simulink model "pos_dvig"  (R2012b)
settings: Solver=ode23tb  StartTime=0.0  StopTime=10  RelTol=1e-3
values from neighbouring files (symbols this model uses):
  J = Jr + Jh    (= 0.0002754438)    [Parameters.m]
  k = 1/(3*R)    (= 0.537634408602)    [Parameters.m]
  ki = 25.5e-3*1/2    (= 0.01275)    [Parameters.m]
  KV = 374    [Parameters.m]
  kw = 30/(KV*pi)*1/2    (= 0.0127664392854)    [Parameters.m]
  P = 8    [Parameters.m]
  Te = L/R    (= 0.000451612903226)    [Parameters.m]
  U = 12    [Parameters.m]
undefined symbols (not defined in the file or in its folder): trapezoid
libraries: simulink x1
settings Model: Creator=botva  LastModifiedBy=botva

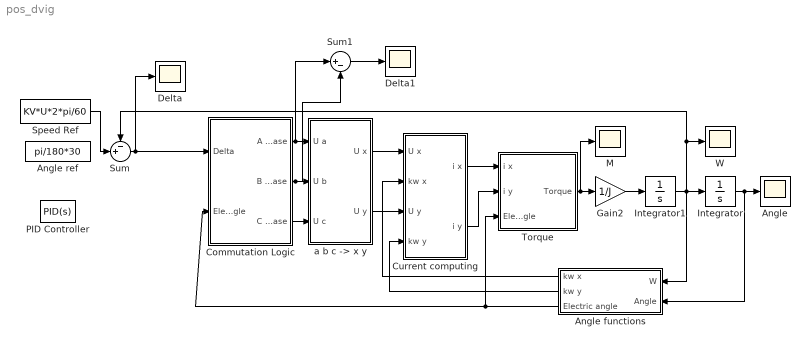
== system pos_dvig ==
  Angle : Scope
      settings: TimeRange=0.06  YMin=-500  YMax=500  DataFormat=Structure
  Angle functions : Subsystem
  Angle ref : Constant  Value=pi/180*30
  Commutation Logic : Subsystem
  Current computing : Subsystem
  Delta : Scope
      settings: TimeRange=0.06  YMin=-500  YMax=500  DataFormat=Structure
  Delta1 : Scope
      settings: TimeRange=0.06  YMin=-12.5  YMax=12.5  SaveName=ScopeData3  DataFormat=Structure
  Gain2 : Gain  Gain=1/J
  Integrator : Integrator
  Integrator1 : Integrator
  M : Scope
      settings: TimeRange=0.06  YMin=-0.025  YMax=0.25  SaveName=ScopeData2  DataFormat=Structure
  PID Controller : simulink/Continuous/PID Controller  Controller=PID  TimeDomain=Continuous-time  SampleTime=1  IntegratorMethod=Forward Euler  FilterMethod=Forward Euler  Form=Parallel  P=0.123357811480852  I=0.544614803683012  D=0.00224722047388112  N=3018.52790886393  InitialConditionSource=internal  InitialConditionForIntegrator=0  InitialConditionForFilter=0  ExternalReset=none  LimitOutput=off  UpperSaturationLimit=inf  LowerSaturationLimit=-inf  LinearizeAsGain=on  AntiWindupMode=none  Kb=1  TrackingMode=off  Kt=1  PParamMin=[]  PParamMax=[]  IParamMin=[]  IParamMax=[]  DParamMin=[]  DParamMax=[]  NParamMin=[]  NParamMax=[]  KbParamMin=[]  KbParamMax=[]  KtParamMin=[]  KtParamMax=[]  POutMin=[]  POutMax=[]  IOutMin=[]  IOutMax=[]  DOutMin=[]  DOutMax=[]  NOutMin=[]  NOutMax=[]  KbOutMin=[]  KbOutMax=[]  KtOutMin=[]  KtOutMax=[]  IntegratorOutMin=[]  IntegratorOutMax=[]  FilterOutMin=[]  FilterOutMax=[]  SumOutMin=[]  SumOutMax=[]  SumI1OutMin=[]  SumI1OutMax=[]  SumI2OutMin=[]  SumI2OutMax=[]  SumI3OutMin=[]  SumI3OutMax=[]  SumDOutMin=[]  SumDOutMax=[]  SaturationOutMin=[]  SaturationOutMax=[]  IntegratorContinuousStateAttributes=''  IntegratorStateMustResolveToSignalObject=off  IntegratorRTWStateStorageClass=Auto  FilterContinuousStateAttributes=''  FilterStateMustResolveToSignalObject=off  FilterRTWStateStorageClass=Auto
  Speed Ref : Constant  Value=KV*U*2*pi/60
  Sum : Sum  Inputs=-+|
  Sum1 : Sum  Inputs=|+-
  Torque : Subsystem
  W : Scope
      settings: TimeRange=0.06  YMin=469.973  YMax=470  SaveName=ScopeData6  DataFormat=Structure
  "a b c -> x y" : Subsystem
  wires:
  Integrator1/1 -> Angle functions/1(W), W/1, Sum/1, Integrator/1
  Integrator/1 -> Angle/1, Angle functions/2(Angle)
  "a b c -> x y"/1(U x) -> Current computing/1(U x)
  Gain2/1 -> Integrator1/1
  Angle functions/3(Electric angle) -> Torque/3(Electric angle), Commutation Logic/2(Electric angle)
  "a b c -> x y"/2(U y) -> Current computing/3(U y)
  Angle functions/2(kw y) -> Current computing/4(kw y)
  Current computing/1(i x) -> Torque/1(i x)
  Current computing/2(i y) -> Torque/2(i y)
  Torque/1(Torque) -> M/1, Gain2/1
  Angle functions/1(kw x) -> Current computing/2(kw x)
  Sum/1 -> Commutation Logic/1(Delta), Delta/1
  Speed Ref/1 -> Sum/2
  Commutation Logic/1(A phase) -> Sum1/1, "a b c -> x y"/1(U a)
  Commutation Logic/2(B phase) -> Sum1/2, "a b c -> x y"/2(U b)
  Commutation Logic/3(C phase) -> "a b c -> x y"/3(U c)
  Sum1/1 -> Delta1/1

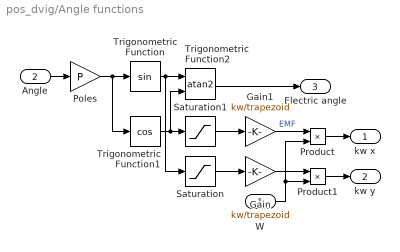
== system pos_dvig/Angle functions ==
  W : Inport
  Angle : Inport  Port=2
  Gain : Gain  Gain=kw/trapezoid
  Gain1 : Gain  Gain=kw/trapezoid
  Poles : Gain  Gain=P
  Product : Product  RndMeth=Zero
  Product1 : Product  RndMeth=Zero
  Saturation : Saturate  UpperLimit=trapezoid  LowerLimit=-trapezoid
  Saturation1 : Saturate  UpperLimit=trapezoid  LowerLimit=-trapezoid
  Trigonometric Function : Trigonometry
  Trigonometric Function1 : Trigonometry  Operator=cos
  Trigonometric Function2 : Trigonometry  Operator=atan2
  kw x : Outport
  kw y : Outport  Port=2
  Electric angle : Outport  Port=3
  wires:
  Trigonometric Function/1 -> Saturation/1, Trigonometric Function2/1
  Trigonometric Function1/1 -> Trigonometric Function2/2, Saturation1/1
  Poles/1 -> Trigonometric Function1/1, Trigonometric Function/1
  Saturation/1 -> Gain/1
  Saturation1/1 -> Gain1/1
  Angle/1 -> Poles/1
  Trigonometric Function2/1 -> Electric angle/1
  Gain1/1 -> Product/1  "EMF"
  Gain/1 -> Product1/1
  Product/1 -> kw x/1
  Product1/1 -> kw y/1
  W/1 -> Product1/2, Product/2

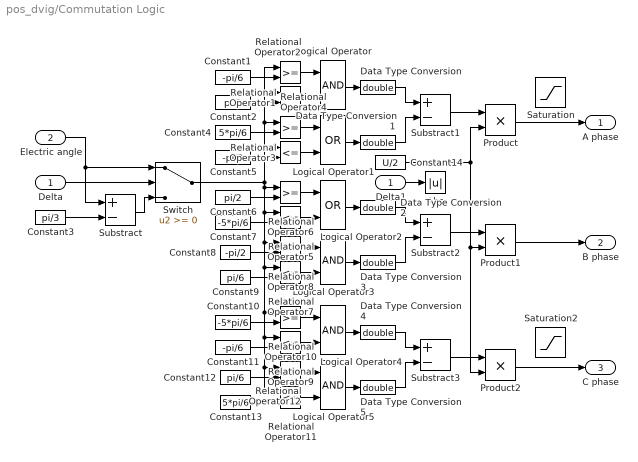
== system pos_dvig/Commutation Logic ==
  Delta : Inport
  Electric angle : Inport  Port=2
  Abs : Abs
  Constant1 : Constant  Value=-pi/6
  Constant10 : Constant  Value=-5*pi/6
  Constant11 : Constant  Value=-pi/6
  Constant12 : Constant  Value=pi/6
  Constant13 : Constant  Value=5*pi/6
  Constant14 : Constant  Value=U/2
  Constant2 : Constant  Value=pi/2
  Constant3 : Constant  Value=pi/3
  Constant4 : Constant  Value=5*pi/6
  Constant5 : Constant  Value=-pi/2
  Constant6 : Constant  Value=pi/2
  Constant7 : Constant  Value=-5*pi/6
  Constant8 : Constant  Value=-pi/2
  Constant9 : Constant  Value=pi/6
  Data Type Conversion{,1..5} (6 alike) : DataTypeConversion  OutDataTypeStr=double
  Delta1 : InportShadow
  Logical Operator{,3..5} (4 alike) : Logic  AllPortsSameDT=off  OutDataTypeStr=boolean
  Logical Operator1 : Logic  Operator=OR  AllPortsSameDT=off  OutDataTypeStr=boolean
  Logical Operator2 : Logic  Operator=OR  AllPortsSameDT=off  OutDataTypeStr=boolean
  Product : Product  RndMeth=Zero
  Product1 : Product  RndMeth=Zero
  Product2 : Product  RndMeth=Zero
  Relational Operator{1,3,5,7,9,11} (6 alike) : RelationalOperator  Operator=<=  InputSameDT=on
  Relational Operator{2,4,6,8,10,12} (6 alike) : RelationalOperator  InputSameDT=on
  Saturation : Saturate  UpperLimit=U  LowerLimit=-U
  Saturation2 : Saturate  UpperLimit=U  LowerLimit=-U
  Substract{,1..3} (4 alike) : Sum  Inputs=+-
  Switch : Switch
  A phase : Outport
  B phase : Outport  Port=2
  C phase : Outport  Port=3
  wires:
  Constant3/1 -> Substract/2
  Substract/1 -> Switch/3
  Electric angle/1 -> Switch/1, Substract/1
  Constant1/1 -> Relational Operator2/2
  Constant2/1 -> Relational Operator1/2
  Relational Operator2/1 -> Logical Operator/1
  Relational Operator1/1 -> Logical Operator/2
  Constant4/1 -> Relational Operator4/2
  Constant5/1 -> Relational Operator3/2
  Relational Operator4/1 -> Logical Operator1/1
  Relational Operator3/1 -> Logical Operator1/2
  Logical Operator/1 -> Data Type Conversion/1
  Logical Operator1/1 -> Data Type Conversion1/1
  Constant6/1 -> Relational Operator6/2
  Constant7/1 -> Relational Operator5/2
  Relational Operator6/1 -> Logical Operator2/1
  Relational Operator5/1 -> Logical Operator2/2
  Constant8/1 -> Relational Operator8/2
  Constant9/1 -> Relational Operator7/2
  Relational Operator8/1 -> Logical Operator3/1
  Relational Operator7/1 -> Logical Operator3/2
  Constant10/1 -> Relational Operator10/2
  Constant11/1 -> Relational Operator9/2
  Relational Operator9/1 -> Logical Operator4/2
  Constant12/1 -> Relational Operator12/2
  Constant13/1 -> Relational Operator11/2
  Relational Operator12/1 -> Logical Operator5/1
  Relational Operator11/1 -> Logical Operator5/2
  Switch/1 -> Relational Operator10/1, Relational Operator11/1, Relational Operator12/1, Relational Operator9/1, Relational Operator7/1, Relational Operator8/1, Relational Operator5/1, Relational Operator6/1, Relational Operator2/1, Relational Operator1/1, Relational Operator4/1, Relational Operator3/1
  Logical Operator4/1 -> Data Type Conversion4/1
  Logical Operator5/1 -> Data Type Conversion5/1
  Relational Operator10/1 -> Logical Operator4/1
  Substract1/1 -> Product/1
  Substract3/1 -> Product2/1
  Substract2/1 -> Product1/1
  Logical Operator2/1 -> Data Type Conversion2/1
  Data Type Conversion/1 -> Substract1/1
  Data Type Conversion1/1 -> Substract1/2
  Data Type Conversion2/1 -> Substract2/1
  Logical Operator3/1 -> Data Type Conversion3/1
  Data Type Conversion3/1 -> Substract2/2
  Data Type Conversion4/1 -> Substract3/1
  Data Type Conversion5/1 -> Substract3/2
  Constant14/1 -> Product2/2, Product1/2, Product/2
  Delta/1 -> Switch/2
  Product/1 -> A phase/1
  Product1/1 -> B phase/1
  Product2/1 -> C phase/1
  Delta1/1 -> Abs/1

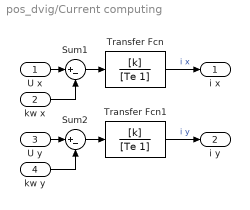
== system pos_dvig/Current computing ==
  U x : Inport
  kw x : Inport  Port=2
  U y : Inport  Port=3
  kw y : Inport  Port=4
  Sum1 : Sum  Inputs=|+-
  Sum2 : Sum  Inputs=|+-
  Transfer Fcn : TransferFcn  Numerator=[k]  Denominator=[Te 1]
  Transfer Fcn1 : TransferFcn  Numerator=[k]  Denominator=[Te 1]
  i x : Outport
  i y : Outport  Port=2
  wires:
  U y/1 -> Sum2/1
  Sum1/1 -> Transfer Fcn/1
  Sum2/1 -> Transfer Fcn1/1
  Transfer Fcn/1 -> i x/1  "i x"
  Transfer Fcn1/1 -> i y/1  "i y"
  kw x/1 -> Sum1/2
  kw y/1 -> Sum2/2
  U x/1 -> Sum1/1

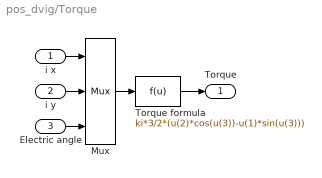
== system pos_dvig/Torque ==
  i x : Inport
  i y : Inport  Port=2
  Electric angle : Inport  Port=3
  Mux : Mux  Inputs=3
  Torque formula : Fcn  Expr=ki*3/2*(u(2)*cos(u(3))-u(1)*sin(u(3)))
  Torque : Outport
  wires:
  i x/1 -> Mux/1
  i y/1 -> Mux/2
  Electric angle/1 -> Mux/3
  Mux/1 -> Torque formula/1
  Torque formula/1 -> Torque/1

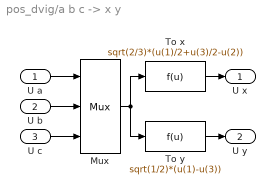
== system pos_dvig/a b c -> x y ==
  U a : Inport
  U b : Inport  Port=2
  U c : Inport  Port=3
  Mux : Mux  Inputs=3
  To x : Fcn  Expr=sqrt(2/3)*(u(1)/2+u(3)/2-u(2))
  To y : Fcn  Expr=sqrt(1/2)*(u(1)-u(3))
  U x : Outport
  U y : Outport  Port=2
  wires:
  U b/1 -> Mux/2
  U c/1 -> Mux/3
  U a/1 -> Mux/1
  Mux/1 -> To y/1, To x/1
  To x/1 -> U x/1
  To y/1 -> U y/1
